simulink library "sm_aileron_actuator_mech_lib"  (R2019a)
settings: Solver=ode45  StartTime=0.0  StopTime=10.0  RelTol=1e-3
undefined symbols (not defined in the file): AAC_Param, actbase_x, actbase_y, smiData, X, Y, Z
libraries: sm_lib x600, fl_lib x3
(part 2 of 12)

== system sm_aileron_actuator_mech_lib/Aileron_Att_1/MountR_Att_1/Bracket C ==
  AilBrk_C_1_RIGID : Subsystem
  Bolt CBrk : Subsystem
  Screws CBrk : Subsystem
  Ail : PMIOPort  Side=Right
  Act : PMIOPort  Port=2  Side=Left
  connections:
  AilBrk_C_1_RIGID/LConn2 -- Act/RConn1
  AilBrk_C_1_RIGID/RConn1 -- Ail/RConn1
  Bolt CBrk/LConn1 -- Screws CBrk/LConn1 -- AilBrk_C_1_RIGID/LConn1

== system sm_aileron_actuator_mech_lib/Aileron_Att_1/MountR_Att_1/Bracket L ==
  AilBrk_L_1_RIGID : Subsystem
  Bolt LBrk : Subsystem
  Screws LBrk : Subsystem
  Ail : PMIOPort  Side=Right
  connections:
  AilBrk_L_1_RIGID/RConn1 -- Ail/RConn1
  Bolt LBrk/LConn1 -- AilBrk_L_1_RIGID/LConn1 -- Screws LBrk/LConn1

== system sm_aileron_actuator_mech_lib/Aileron_Att_1/MountR_Att_1/Bracket R ==
  AilBrk_R_1_RIGID : Subsystem
  Bolt RBrk : Subsystem
  Screws RBrk : Subsystem
  Ail : PMIOPort  Side=Right
  connections:
  AilBrk_R_1_RIGID/RConn1 -- Ail/RConn1
  Bolt RBrk/LConn1 -- AilBrk_R_1_RIGID/LConn1 -- Screws RBrk/LConn1

== system sm_aileron_actuator_mech_lib/Aileron Mech/Aileron_Att_1/MountC_Att_1/Bracket C ==
  AilBrk_C_1_RIGID : Subsystem
  Bolt CBrk : Subsystem
  Screws CBrk : Subsystem
  Ail : PMIOPort  Side=Right
  Act : PMIOPort  Port=2  Side=Left
  connections:
  AilBrk_C_1_RIGID/LConn1 -- Screws CBrk/LConn1 -- Bolt CBrk/LConn1
  AilBrk_C_1_RIGID/RConn1 -- Ail/RConn1
  AilBrk_C_1_RIGID/LConn2 -- Act/RConn1

== system sm_aileron_actuator_mech_lib/Aileron Mech/Aileron_Att_1/MountC_Att_1/Bracket L ==
  AilBrk_L_1_RIGID : Subsystem
  Bolt LBrk : Subsystem
  Screws LBrk : Subsystem
  M : PMIOPort  Side=Left
  Ail : PMIOPort  Port=2  Side=Right
  connections:
  Screws LBrk/LConn1 -- Bolt LBrk/LConn2 -- AilBrk_L_1_RIGID/LConn1
  Bolt LBrk/LConn1 -- M/RConn1
  AilBrk_L_1_RIGID/RConn1 -- Ail/RConn1

== system sm_aileron_actuator_mech_lib/Aileron Mech/Aileron_Att_1/MountC_Att_1/Bracket R ==
  AilBrk_R_1_RIGID : Subsystem
  Bolt RBrk : Subsystem
  Screws RBrk : Subsystem
  Ail : PMIOPort  Side=Right
  connections:
  AilBrk_R_1_RIGID/LConn1 -- Screws RBrk/LConn1 -- Bolt RBrk/LConn1
  AilBrk_R_1_RIGID/RConn1 -- Ail/RConn1

== system sm_aileron_actuator_mech_lib/Aileron Mech/Aileron_Att_1/MountL_Att_1/Bracket C ==
  AilBrk_C_1_RIGID : Subsystem
  Bolt CBrk : Subsystem
  Screws CBrk : Subsystem
  Ail : PMIOPort  Side=Right
  Act : PMIOPort  Port=2  Side=Left
  connections:
  AilBrk_C_1_RIGID/LConn1 -- Screws CBrk/LConn1 -- Bolt CBrk/LConn1
  AilBrk_C_1_RIGID/LConn2 -- Act/RConn1
  AilBrk_C_1_RIGID/RConn1 -- Ail/RConn1

== system sm_aileron_actuator_mech_lib/Aileron Mech/Aileron_Att_1/MountL_Att_1/Bracket L ==
  AilBrk_L_1_RIGID : Subsystem
  Bolt LBrk : Subsystem
  "Screws LBrk " : Subsystem
  Ail : PMIOPort  Side=Right
  connections:
  AilBrk_L_1_RIGID/LConn1 -- "Screws LBrk "/LConn1 -- Bolt LBrk/LConn1
  AilBrk_L_1_RIGID/RConn1 -- Ail/RConn1

== system sm_aileron_actuator_mech_lib/Aileron Mech/Aileron_Att_1/MountL_Att_1/Bracket R ==
  AilBrk_R_1_RIGID : Subsystem
  Bolt RBrk : Subsystem
  Screws RBrk : Subsystem
  Ail : PMIOPort  Side=Right
  connections:
  AilBrk_R_1_RIGID/LConn1 -- Screws RBrk/LConn1 -- Bolt RBrk/LConn1
  AilBrk_R_1_RIGID/RConn1 -- Ail/RConn1

== system sm_aileron_actuator_mech_lib/Aileron Mech/Aileron_Att_1/MountR_Att_1/Bracket C ==
  AilBrk_C_1_RIGID : Subsystem
  Bolt CBrk : Subsystem
  Screws CBrk : Subsystem
  Ail : PMIOPort  Side=Right
  Act : PMIOPort  Port=2  Side=Left
  connections:
  AilBrk_C_1_RIGID/LConn1 -- Screws CBrk/LConn1 -- Bolt CBrk/LConn1
  AilBrk_C_1_RIGID/RConn1 -- Ail/RConn1
  AilBrk_C_1_RIGID/LConn2 -- Act/RConn1

== system sm_aileron_actuator_mech_lib/Aileron Mech/Aileron_Att_1/MountR_Att_1/Bracket L ==
  AilBrk_L_1_RIGID : Subsystem
  Bolt LBrk : Subsystem
  Screws LBrk : Subsystem
  Ail : PMIOPort  Side=Right
  connections:
  Screws LBrk/LConn1 -- AilBrk_L_1_RIGID/LConn1 -- Bolt LBrk/LConn1
  AilBrk_L_1_RIGID/RConn1 -- Ail/RConn1

== system sm_aileron_actuator_mech_lib/Aileron Mech/Aileron_Att_1/MountR_Att_1/Bracket R ==
  AilBrk_R_1_RIGID : Subsystem
  Bolt RBrk : Subsystem
  Screws RBrk : Subsystem
  Ail : PMIOPort  Side=Right
  connections:
  Screws RBrk/LConn1 -- AilBrk_R_1_RIGID/LConn1 -- Bolt RBrk/LConn1
  AilBrk_R_1_RIGID/RConn1 -- Ail/RConn1

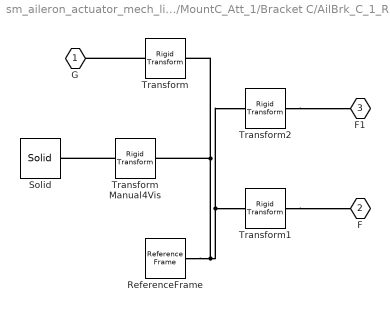
== system sm_aileron_actuator_mech_lib/Aileron_Att_1/MountC_Att_1/Bracket C/AilBrk_C_1_RIGID ==
  ReferenceFrame : sm_lib/Frames and Transforms/Reference Frame
  Solid : sm_lib/Body Elements/Solid  InertiaType=Custom  Mass=smiData.Solid(15).mass  MassUnits=kg  CenterOfMass=smiData.Solid(15).CoM  CenterOfMassUnits=m  MomentsOfInertia=smiData.Solid(15).MoI  MomentsOfInertiaUnits=kg*m^2  ProductsOfInertia=smiData.Solid(15).PoI  ProductsOfInertiaUnits=kg*m^2  BasedOnType=Density  Density=1000  DensityUnits=kg/m^3  DoExposeReferenceFrame=on  SerializedFrames=<Frames/>  GraphicType=FromGeometry  MarkerShape=Sphere  MarkerSize=10  GraphicVisPropType=SimpleVisualProperties  GraphicDiffuseColor=smiData.Solid(15).color  GraphicSpecularColor=[0.5 0.5 0.5 1.0]  GraphicAmbientColor=[0.15 0.15 0.15 1.0]  GraphicEmissiveColor=[0.0 0.0 0.0 1.0]  GraphicShininess=75  GraphicOpacity=smiData.Solid(15).opacity  GeometryShape=FromFile  RectangleSize=[1 1]  RectangleSizeUnits=m  BrickDimensions=[1 1 1]  BrickDimensionUnits=m  CylinderRadius=1  CylinderRadiusUnits=m  CylinderLength=1  CylinderLengthUnits=m  SphereRadius=1  SphereRadiusUnits=m  EllipsoidRadii=[1 1 1]  EllipsoidRadiiUnits=m  ExtrusionCrossSection=[1 1; -1 1; -1 -1; 1 -1]  ExtrusionCrossSectionUnits=m  ExtrusionLength=1  ExtrusionLengthUnits=m  PolygonNumSides=3  PolygonOuterRadius=1  PolygonOuterRadiusUnits=m  ExtGeomFileType=STEP  ExtGeomFileName=AilBrk_C.step  ExtGeomFileUnits=m  RevolutionCrossSection=[1 1; 1 -1; 2 -1; 2 1]  RevolutionCrossSectionUnits=m  RevolutionExtent=Full  RevolutionAngle=180  RevolutionAngleUnits=deg
  Transform : sm_lib/Frames and Transforms/Rigid Transform  TranslationMethod=Cartesian  TranslationStandardOffset=0  TranslationLengthUnit=m  TranslationStandardAxis=+Z  TranslationCartesianOffset=smiData.RigidTransform(98).translation  TranslationROffset=0  TranslationROffsetUnits=m  TranslationZOffset=0  TranslationZOffsetUnits=m  TranslationThetaOffset=0  TranslationThetaOffsetUnits=deg  RotationMethod=ArbitraryAxis  RotationAngleUnits=rad  RotationStandardAxis=+Z  RotationAngle=smiData.RigidTransform(98).angle  RotationArbitraryAxis=smiData.RigidTransform(98).axis  FollAlignAxisA=+X  BaseAlignAxisA=+Y  FollAlignAxisB=+Y  BaseAlignAxisB=+Z  RotationSequenceAxes=FollowerAxes  RotationSequence=XYX  RotationSequenceAngles=[0 0 0]  RotationSequenceAnglesUnits=deg  RotationMatrix=[1 0 0; 0 1 0; 0 0 1]
  Transform Manual4Vis : sm_lib/Frames and Transforms/Rigid Transform  TranslationMethod=Cartesian  TranslationStandardOffset=0  TranslationLengthUnit=m  TranslationStandardAxis=+Z  TranslationCartesianOffset=[-1 1 0]*AAC_Param.AilBrk.LRManual4Vis  TranslationROffset=0  TranslationROffsetUnits=m  TranslationZOffset=0  TranslationZOffsetUnits=m  TranslationThetaOffset=0  TranslationThetaOffsetUnits=deg  RotationMethod=None  RotationAngleUnits=deg  RotationStandardAxis=+Z  RotationAngle=0.0  RotationArbitraryAxis=[0 0 1]  FollAlignAxisA=+X  BaseAlignAxisA=+Y  FollAlignAxisB=+Y  BaseAlignAxisB=+Z  RotationSequenceAxes=FollowerAxes  RotationSequence=XYX  RotationSequenceAngles=[0 0 0]  RotationSequenceAnglesUnits=deg  RotationMatrix=[1 0 0; 0 1 0; 0 0 1]
  Transform1 : sm_lib/Frames and Transforms/Rigid Transform  TranslationMethod=Cartesian  TranslationStandardOffset=0  TranslationLengthUnit=m  TranslationStandardAxis=+Z  TranslationCartesianOffset=smiData.RigidTransform(172).translation  TranslationROffset=0  TranslationROffsetUnits=m  TranslationZOffset=0  TranslationZOffsetUnits=m  TranslationThetaOffset=0  TranslationThetaOffsetUnits=deg  RotationMethod=ArbitraryAxis  RotationAngleUnits=rad  RotationStandardAxis=+Z  RotationAngle=smiData.RigidTransform(172).angle  RotationArbitraryAxis=smiData.RigidTransform(172).axis  FollAlignAxisA=+X  BaseAlignAxisA=+Y  FollAlignAxisB=+Y  BaseAlignAxisB=+Z  RotationSequenceAxes=FollowerAxes  RotationSequence=XYX  RotationSequenceAngles=[0 0 0]  RotationSequenceAnglesUnits=deg  RotationMatrix=[1 0 0; 0 1 0; 0 0 1]
  Transform2 : sm_lib/Frames and Transforms/Rigid Transform  TranslationMethod=Cartesian  TranslationStandardOffset=0  TranslationLengthUnit=m  TranslationStandardAxis=+Z  TranslationCartesianOffset=smiData.RigidTransform(200).translation  TranslationROffset=0  TranslationROffsetUnits=m  TranslationZOffset=0  TranslationZOffsetUnits=m  TranslationThetaOffset=0  TranslationThetaOffsetUnits=deg  RotationMethod=ArbitraryAxis  RotationAngleUnits=rad  RotationStandardAxis=+Z  RotationAngle=smiData.RigidTransform(200).angle  RotationArbitraryAxis=smiData.RigidTransform(200).axis  FollAlignAxisA=+X  BaseAlignAxisA=+Y  FollAlignAxisB=+Y  BaseAlignAxisB=+Z  RotationSequenceAxes=FollowerAxes  RotationSequence=XYX  RotationSequenceAngles=[0 0 0]  RotationSequenceAnglesUnits=deg  RotationMatrix=[1 0 0; 0 1 0; 0 0 1]
  G : PMIOPort  Side=Left
  F : PMIOPort  Port=2  Side=Right
  F1 : PMIOPort  Port=3  Side=Left
  connections:
  Transform/RConn1 -- Transform Manual4Vis/LConn1 -- Transform2/LConn1 -- Transform1/LConn1 -- ReferenceFrame/RConn1
  Transform2/RConn1 -- F1/RConn1
  Transform1/RConn1 -- F/RConn1
  Transform/LConn1 -- G/RConn1
  Transform Manual4Vis/RConn1 -- Solid/RConn1

== system sm_aileron_actuator_mech_lib/Aileron_Att_1/MountC_Att_1/Bracket C/Bolt CBrk ==
  Hex_Flange_Screw_M6_1_RIGID : Subsystem
  Hex_Flange_Screw_M6_2_RIGID : Subsystem
  Hex_Flange_Screw_M6_3_RIGID : Subsystem
  Hex_Flange_Screw_M6_4_RIGID : Subsystem
  Hex_Flange_Screw_M6_5_RIGID : Subsystem
  Hex_Flange_Screw_M6_6_RIGID : Subsystem
  G : PMIOPort  Side=Left
  connections:
  Hex_Flange_Screw_M6_4_RIGID/LConn1 -- Hex_Flange_Screw_M6_3_RIGID/LConn1 -- Hex_Flange_Screw_M6_2_RIGID/LConn1 -- Hex_Flange_Screw_M6_1_RIGID/LConn1 -- G/RConn1 -- Hex_Flange_Screw_M6_5_RIGID/LConn1 -- Hex_Flange_Screw_M6_6_RIGID/LConn1

== system sm_aileron_actuator_mech_lib/Aileron_Att_1/MountC_Att_1/Bracket C/Screws CBrk ==
  Hex_Bolt_M10_3_RIGID : Subsystem
  Hex_Flange_Nut_M10_1_RIGID : Subsystem
  Washer_3_RIGID : Subsystem
  Washer_4_RIGID : Subsystem
  G : PMIOPort  Side=Left
  connections:
  Hex_Flange_Nut_M10_1_RIGID/LConn1 -- Washer_3_RIGID/LConn1 -- Washer_4_RIGID/LConn1 -- G/RConn1 -- Hex_Bolt_M10_3_RIGID/LConn1

== system sm_aileron_actuator_mech_lib/Aileron_Att_1/MountC_Att_1/Bracket L/AilBrk_L_1_RIGID ==
  ReferenceFrame : sm_lib/Frames and Transforms/Reference Frame
  Solid : sm_lib/Body Elements/Solid  InertiaType=Custom  Mass=smiData.Solid(13).mass  MassUnits=kg  CenterOfMass=smiData.Solid(13).CoM  CenterOfMassUnits=m  MomentsOfInertia=smiData.Solid(13).MoI  MomentsOfInertiaUnits=kg*m^2  ProductsOfInertia=smiData.Solid(13).PoI  ProductsOfInertiaUnits=kg*m^2  BasedOnType=Density  Density=1000  DensityUnits=kg/m^3  DoExposeReferenceFrame=on  SerializedFrames=<Frames/>  GraphicType=FromGeometry  MarkerShape=Sphere  MarkerSize=10  GraphicVisPropType=SimpleVisualProperties  GraphicDiffuseColor=smiData.Solid(13).color  GraphicSpecularColor=[0.5 0.5 0.5 1.0]  GraphicAmbientColor=[0.15 0.15 0.15 1.0]  GraphicEmissiveColor=[0.0 0.0 0.0 1.0]  GraphicShininess=75  GraphicOpacity=smiData.Solid(13).opacity  GeometryShape=FromFile  RectangleSize=[1 1]  RectangleSizeUnits=m  BrickDimensions=[1 1 1]  BrickDimensionUnits=m  CylinderRadius=1  CylinderRadiusUnits=m  CylinderLength=1  CylinderLengthUnits=m  SphereRadius=1  SphereRadiusUnits=m  EllipsoidRadii=[1 1 1]  EllipsoidRadiiUnits=m  ExtrusionCrossSection=[1 1; -1 1; -1 -1; 1 -1]  ExtrusionCrossSectionUnits=m  ExtrusionLength=1  ExtrusionLengthUnits=m  PolygonNumSides=3  PolygonOuterRadius=1  PolygonOuterRadiusUnits=m  ExtGeomFileType=STEP  ExtGeomFileName=AilBrk_L.step  ExtGeomFileUnits=m  RevolutionCrossSection=[1 1; 1 -1; 2 -1; 2 1]  RevolutionCrossSectionUnits=m  RevolutionExtent=Full  RevolutionAngle=180  RevolutionAngleUnits=deg
  Transform : sm_lib/Frames and Transforms/Rigid Transform  TranslationMethod=Cartesian  TranslationStandardOffset=0  TranslationLengthUnit=m  TranslationStandardAxis=+Z  TranslationCartesianOffset=smiData.RigidTransform(103).translation  TranslationROffset=0  TranslationROffsetUnits=m  TranslationZOffset=0  TranslationZOffsetUnits=m  TranslationThetaOffset=0  TranslationThetaOffsetUnits=deg  RotationMethod=ArbitraryAxis  RotationAngleUnits=rad  RotationStandardAxis=+Z  RotationAngle=smiData.RigidTransform(103).angle  RotationArbitraryAxis=smiData.RigidTransform(103).axis  FollAlignAxisA=+X  BaseAlignAxisA=+Y  FollAlignAxisB=+Y  BaseAlignAxisB=+Z  RotationSequenceAxes=FollowerAxes  RotationSequence=XYX  RotationSequenceAngles=[0 0 0]  RotationSequenceAnglesUnits=deg  RotationMatrix=[1 0 0; 0 1 0; 0 0 1]
  Transform Manual4Vis : sm_lib/Frames and Transforms/Rigid Transform  TranslationMethod=StandardAxis  TranslationStandardOffset=AAC_Param.AilBrk.LRManual4Vis  TranslationLengthUnit=m  TranslationStandardAxis=+Y  TranslationCartesianOffset=[0 0 0]  TranslationROffset=0  TranslationROffsetUnits=m  TranslationZOffset=0  TranslationZOffsetUnits=m  TranslationThetaOffset=0  TranslationThetaOffsetUnits=deg  RotationMethod=None  RotationAngleUnits=deg  RotationStandardAxis=+Z  RotationAngle=0.0  RotationArbitraryAxis=[0 0 1]  FollAlignAxisA=+X  BaseAlignAxisA=+Y  FollAlignAxisB=+Y  BaseAlignAxisB=+Z  RotationSequenceAxes=FollowerAxes  RotationSequence=XYX  RotationSequenceAngles=[0 0 0]  RotationSequenceAnglesUnits=deg  RotationMatrix=[1 0 0; 0 1 0; 0 0 1]
  Transform1 : sm_lib/Frames and Transforms/Rigid Transform  TranslationMethod=Cartesian  TranslationStandardOffset=0  TranslationLengthUnit=m  TranslationStandardAxis=+Z  TranslationCartesianOffset=smiData.RigidTransform(174).translation  TranslationROffset=0  TranslationROffsetUnits=m  TranslationZOffset=0  TranslationZOffsetUnits=m  TranslationThetaOffset=0  TranslationThetaOffsetUnits=deg  RotationMethod=ArbitraryAxis  RotationAngleUnits=rad  RotationStandardAxis=+Z  RotationAngle=smiData.RigidTransform(174).angle  RotationArbitraryAxis=smiData.RigidTransform(174).axis  FollAlignAxisA=+X  BaseAlignAxisA=+Y  FollAlignAxisB=+Y  BaseAlignAxisB=+Z  RotationSequenceAxes=FollowerAxes  RotationSequence=XYX  RotationSequenceAngles=[0 0 0]  RotationSequenceAnglesUnits=deg  RotationMatrix=[1 0 0; 0 1 0; 0 0 1]
  G : PMIOPort  Side=Left
  F : PMIOPort  Port=2  Side=Right
  connections:
  Transform Manual4Vis/RConn1 -- Solid/RConn1
  Transform1/RConn1 -- F/RConn1
  Transform/LConn1 -- G/RConn1
  Transform/RConn1 -- Transform1/LConn1 -- ReferenceFrame/RConn1 -- Transform Manual4Vis/LConn1

== system sm_aileron_actuator_mech_lib/Aileron_Att_1/MountC_Att_1/Bracket L/Bolt LBrk ==
  Hex_Bolt_M10_2_RIGID : Subsystem
  Washer_1_RIGID : Subsystem
  M : PMIOPort  Side=Left
  G : PMIOPort  Port=2  Side=Left
  connections:
  Washer_1_RIGID/LConn1 -- M/RConn1
  G/RConn1 -- Hex_Bolt_M10_2_RIGID/LConn1 -- Washer_1_RIGID/LConn2

== system sm_aileron_actuator_mech_lib/Aileron_Att_1/MountC_Att_1/Bracket L/Screws LBrk ==
  Oval_Head_M4_12_RIGID : Subsystem
  Oval_Head_M4_1_RIGID : Subsystem
  Oval_Head_M4_4_RIGID : Subsystem
  Oval_Head_M4_5_RIGID : Subsystem
  Oval_Head_M4_6_RIGID : Subsystem
  Oval_Head_M4_8_RIGID : Subsystem
  G : PMIOPort  Side=Left
  connections:
  Oval_Head_M4_12_RIGID/LConn1 -- Oval_Head_M4_4_RIGID/LConn1 -- Oval_Head_M4_5_RIGID/LConn1 -- Oval_Head_M4_6_RIGID/LConn1 -- Oval_Head_M4_8_RIGID/LConn1 -- G/RConn1 -- Oval_Head_M4_1_RIGID/LConn1

== system sm_aileron_actuator_mech_lib/Aileron_Att_1/MountC_Att_1/Bracket R/AilBrk_R_1_RIGID ==
  ReferenceFrame : sm_lib/Frames and Transforms/Reference Frame
  Solid : sm_lib/Body Elements/Solid  InertiaType=Custom  Mass=smiData.Solid(16).mass  MassUnits=kg  CenterOfMass=smiData.Solid(16).CoM  CenterOfMassUnits=m  MomentsOfInertia=smiData.Solid(16).MoI  MomentsOfInertiaUnits=kg*m^2  ProductsOfInertia=smiData.Solid(16).PoI  ProductsOfInertiaUnits=kg*m^2  BasedOnType=Density  Density=1000  DensityUnits=kg/m^3  DoExposeReferenceFrame=on  SerializedFrames=<Frames/>  GraphicType=FromGeometry  MarkerShape=Sphere  MarkerSize=10  GraphicVisPropType=SimpleVisualProperties  GraphicDiffuseColor=smiData.Solid(16).color  GraphicSpecularColor=[0.5 0.5 0.5 1.0]  GraphicAmbientColor=[0.15 0.15 0.15 1.0]  GraphicEmissiveColor=[0.0 0.0 0.0 1.0]  GraphicShininess=75  GraphicOpacity=smiData.Solid(16).opacity  GeometryShape=FromFile  RectangleSize=[1 1]  RectangleSizeUnits=m  BrickDimensions=[1 1 1]  BrickDimensionUnits=m  CylinderRadius=1  CylinderRadiusUnits=m  CylinderLength=1  CylinderLengthUnits=m  SphereRadius=1  SphereRadiusUnits=m  EllipsoidRadii=[1 1 1]  EllipsoidRadiiUnits=m  ExtrusionCrossSection=[1 1; -1 1; -1 -1; 1 -1]  ExtrusionCrossSectionUnits=m  ExtrusionLength=1  ExtrusionLengthUnits=m  PolygonNumSides=3  PolygonOuterRadius=1  PolygonOuterRadiusUnits=m  ExtGeomFileType=STEP  ExtGeomFileName=AilBrk_R.step  ExtGeomFileUnits=m  RevolutionCrossSection=[1 1; 1 -1; 2 -1; 2 1]  RevolutionCrossSectionUnits=m  RevolutionExtent=Full  RevolutionAngle=180  RevolutionAngleUnits=deg
  Transform : sm_lib/Frames and Transforms/Rigid Transform  TranslationMethod=Cartesian  TranslationStandardOffset=0  TranslationLengthUnit=m  TranslationStandardAxis=+Z  TranslationCartesianOffset=smiData.RigidTransform(82).translation  TranslationROffset=0  TranslationROffsetUnits=m  TranslationZOffset=0  TranslationZOffsetUnits=m  TranslationThetaOffset=0  TranslationThetaOffsetUnits=deg  RotationMethod=ArbitraryAxis  RotationAngleUnits=rad  RotationStandardAxis=+Z  RotationAngle=smiData.RigidTransform(82).angle  RotationArbitraryAxis=smiData.RigidTransform(82).axis  FollAlignAxisA=+X  BaseAlignAxisA=+Y  FollAlignAxisB=+Y  BaseAlignAxisB=+Z  RotationSequenceAxes=FollowerAxes  RotationSequence=XYX  RotationSequenceAngles=[0 0 0]  RotationSequenceAnglesUnits=deg  RotationMatrix=[1 0 0; 0 1 0; 0 0 1]
  Transform Manual4Vis : sm_lib/Frames and Transforms/Rigid Transform  TranslationMethod=StandardAxis  TranslationStandardOffset=AAC_Param.AilBrk.LRManual4Vis  TranslationLengthUnit=m  TranslationStandardAxis=-Y  TranslationCartesianOffset=[0 0 0]  TranslationROffset=0  TranslationROffsetUnits=m  TranslationZOffset=0  TranslationZOffsetUnits=m  TranslationThetaOffset=0  TranslationThetaOffsetUnits=deg  RotationMethod=None  RotationAngleUnits=deg  RotationStandardAxis=+Z  RotationAngle=0.0  RotationArbitraryAxis=[0 0 1]  FollAlignAxisA=+X  BaseAlignAxisA=+Y  FollAlignAxisB=+Y  BaseAlignAxisB=+Z  RotationSequenceAxes=FollowerAxes  RotationSequence=XYX  RotationSequenceAngles=[0 0 0]  RotationSequenceAnglesUnits=deg  RotationMatrix=[1 0 0; 0 1 0; 0 0 1]
  Transform1 : sm_lib/Frames and Transforms/Rigid Transform  TranslationMethod=Cartesian  TranslationStandardOffset=0  TranslationLengthUnit=m  TranslationStandardAxis=+Z  TranslationCartesianOffset=smiData.RigidTransform(176).translation  TranslationROffset=0  TranslationROffsetUnits=m  TranslationZOffset=0  TranslationZOffsetUnits=m  TranslationThetaOffset=0  TranslationThetaOffsetUnits=deg  RotationMethod=ArbitraryAxis  RotationAngleUnits=rad  RotationStandardAxis=+Z  RotationAngle=smiData.RigidTransform(176).angle  RotationArbitraryAxis=smiData.RigidTransform(176).axis  FollAlignAxisA=+X  BaseAlignAxisA=+Y  FollAlignAxisB=+Y  BaseAlignAxisB=+Z  RotationSequenceAxes=FollowerAxes  RotationSequence=XYX  RotationSequenceAngles=[0 0 0]  RotationSequenceAnglesUnits=deg  RotationMatrix=[1 0 0; 0 1 0; 0 0 1]
  G : PMIOPort  Side=Left
  F : PMIOPort  Port=2  Side=Right
  connections:
  Transform Manual4Vis/RConn1 -- Solid/RConn1
  Transform1/RConn1 -- F/RConn1
  Transform/LConn1 -- G/RConn1
  Transform/RConn1 -- Transform1/LConn1 -- ReferenceFrame/RConn1 -- Transform Manual4Vis/LConn1

== system sm_aileron_actuator_mech_lib/Aileron_Att_1/MountC_Att_1/Bracket R/Bolt RBrk ==
  Hex_Bolt_M10_1_RIGID : Subsystem
  Washer_2_RIGID : Subsystem
  G : PMIOPort  Side=Left
  connections:
  Washer_2_RIGID/LConn1 -- G/RConn1 -- Hex_Bolt_M10_1_RIGID/LConn1

== system sm_aileron_actuator_mech_lib/Aileron_Att_1/MountC_Att_1/Bracket R/Screws RBrk ==
  Oval_Head_M4_10_RIGID : Subsystem
  Oval_Head_M4_11_RIGID : Subsystem
  Oval_Head_M4_2_RIGID : Subsystem
  Oval_Head_M4_3_RIGID : Subsystem
  Oval_Head_M4_7_RIGID : Subsystem
  Oval_Head_M4_9_RIGID : Subsystem
  G : PMIOPort  Side=Left
  connections:
  Oval_Head_M4_7_RIGID/LConn1 -- Oval_Head_M4_9_RIGID/LConn1 -- Oval_Head_M4_2_RIGID/LConn1 -- Oval_Head_M4_11_RIGID/LConn1 -- Oval_Head_M4_10_RIGID/LConn1 -- G/RConn1 -- Oval_Head_M4_3_RIGID/LConn1

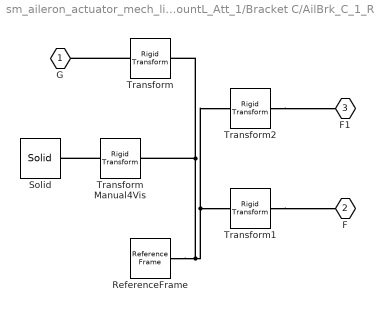
== system sm_aileron_actuator_mech_lib/Aileron_Att_1/MountL_Att_1/Bracket C/AilBrk_C_1_RIGID ==
  ReferenceFrame : sm_lib/Frames and Transforms/Reference Frame
  Solid : sm_lib/Body Elements/Solid  InertiaType=Custom  Mass=smiData.Solid(15).mass  MassUnits=kg  CenterOfMass=smiData.Solid(15).CoM  CenterOfMassUnits=m  MomentsOfInertia=smiData.Solid(15).MoI  MomentsOfInertiaUnits=kg*m^2  ProductsOfInertia=smiData.Solid(15).PoI  ProductsOfInertiaUnits=kg*m^2  BasedOnType=Density  Density=1000  DensityUnits=kg/m^3  DoExposeReferenceFrame=on  SerializedFrames=<Frames/>  GraphicType=FromGeometry  MarkerShape=Sphere  MarkerSize=10  GraphicVisPropType=SimpleVisualProperties  GraphicDiffuseColor=smiData.Solid(15).color  GraphicSpecularColor=[0.5 0.5 0.5 1.0]  GraphicAmbientColor=[0.15 0.15 0.15 1.0]  GraphicEmissiveColor=[0.0 0.0 0.0 1.0]  GraphicShininess=75  GraphicOpacity=smiData.Solid(15).opacity  GeometryShape=FromFile  RectangleSize=[1 1]  RectangleSizeUnits=m  BrickDimensions=[1 1 1]  BrickDimensionUnits=m  CylinderRadius=1  CylinderRadiusUnits=m  CylinderLength=1  CylinderLengthUnits=m  SphereRadius=1  SphereRadiusUnits=m  EllipsoidRadii=[1 1 1]  EllipsoidRadiiUnits=m  ExtrusionCrossSection=[1 1; -1 1; -1 -1; 1 -1]  ExtrusionCrossSectionUnits=m  ExtrusionLength=1  ExtrusionLengthUnits=m  PolygonNumSides=3  PolygonOuterRadius=1  PolygonOuterRadiusUnits=m  ExtGeomFileType=STEP  ExtGeomFileName=AilBrk_C.step  ExtGeomFileUnits=m  RevolutionCrossSection=[1 1; 1 -1; 2 -1; 2 1]  RevolutionCrossSectionUnits=m  RevolutionExtent=Full  RevolutionAngle=180  RevolutionAngleUnits=deg
  Transform : sm_lib/Frames and Transforms/Rigid Transform  TranslationMethod=Cartesian  TranslationStandardOffset=0  TranslationLengthUnit=m  TranslationStandardAxis=+Z  TranslationCartesianOffset=smiData.RigidTransform(161).translation  TranslationROffset=0  TranslationROffsetUnits=m  TranslationZOffset=0  TranslationZOffsetUnits=m  TranslationThetaOffset=0  TranslationThetaOffsetUnits=deg  RotationMethod=ArbitraryAxis  RotationAngleUnits=rad  RotationStandardAxis=+Z  RotationAngle=smiData.RigidTransform(161).angle  RotationArbitraryAxis=smiData.RigidTransform(161).axis  FollAlignAxisA=+X  BaseAlignAxisA=+Y  FollAlignAxisB=+Y  BaseAlignAxisB=+Z  RotationSequenceAxes=FollowerAxes  RotationSequence=XYX  RotationSequenceAngles=[0 0 0]  RotationSequenceAnglesUnits=deg  RotationMatrix=[1 0 0; 0 1 0; 0 0 1]
  Transform Manual4Vis : sm_lib/Frames and Transforms/Rigid Transform  TranslationMethod=Cartesian  TranslationStandardOffset=0  TranslationLengthUnit=m  TranslationStandardAxis=+Z  TranslationCartesianOffset=[-1 1 0]*AAC_Param.AilBrk.LRManual4Vis  TranslationROffset=0  TranslationROffsetUnits=m  TranslationZOffset=0  TranslationZOffsetUnits=m  TranslationThetaOffset=0  TranslationThetaOffsetUnits=deg  RotationMethod=None  RotationAngleUnits=deg  RotationStandardAxis=+Z  RotationAngle=0.0  RotationArbitraryAxis=[0 0 1]  FollAlignAxisA=+X  BaseAlignAxisA=+Y  FollAlignAxisB=+Y  BaseAlignAxisB=+Z  RotationSequenceAxes=FollowerAxes  RotationSequence=XYX  RotationSequenceAngles=[0 0 0]  RotationSequenceAnglesUnits=deg  RotationMatrix=[1 0 0; 0 1 0; 0 0 1]
  Transform1 : sm_lib/Frames and Transforms/Rigid Transform  TranslationMethod=Cartesian  TranslationStandardOffset=0  TranslationLengthUnit=m  TranslationStandardAxis=+Z  TranslationCartesianOffset=smiData.RigidTransform(185).translation  TranslationROffset=0  TranslationROffsetUnits=m  TranslationZOffset=0  TranslationZOffsetUnits=m  TranslationThetaOffset=0  TranslationThetaOffsetUnits=deg  RotationMethod=ArbitraryAxis  RotationAngleUnits=rad  RotationStandardAxis=+Z  RotationAngle=smiData.RigidTransform(185).angle  RotationArbitraryAxis=smiData.RigidTransform(185).axis  FollAlignAxisA=+X  BaseAlignAxisA=+Y  FollAlignAxisB=+Y  BaseAlignAxisB=+Z  RotationSequenceAxes=FollowerAxes  RotationSequence=XYX  RotationSequenceAngles=[0 0 0]  RotationSequenceAnglesUnits=deg  RotationMatrix=[1 0 0; 0 1 0; 0 0 1]
  Transform2 : sm_lib/Frames and Transforms/Rigid Transform  TranslationMethod=Cartesian  TranslationStandardOffset=0  TranslationLengthUnit=m  TranslationStandardAxis=+Z  TranslationCartesianOffset=smiData.RigidTransform(202).translation  TranslationROffset=0  TranslationROffsetUnits=m  TranslationZOffset=0  TranslationZOffsetUnits=m  TranslationThetaOffset=0  TranslationThetaOffsetUnits=deg  RotationMethod=ArbitraryAxis  RotationAngleUnits=rad  RotationStandardAxis=+Z  RotationAngle=smiData.RigidTransform(202).angle  RotationArbitraryAxis=smiData.RigidTransform(202).axis  FollAlignAxisA=+X  BaseAlignAxisA=+Y  FollAlignAxisB=+Y  BaseAlignAxisB=+Z  RotationSequenceAxes=FollowerAxes  RotationSequence=XYX  RotationSequenceAngles=[0 0 0]  RotationSequenceAnglesUnits=deg  RotationMatrix=[1 0 0; 0 1 0; 0 0 1]
  G : PMIOPort  Side=Left
  F : PMIOPort  Port=2  Side=Right
  F1 : PMIOPort  Port=3  Side=Left
  connections:
  Transform Manual4Vis/RConn1 -- Solid/RConn1
  Transform2/RConn1 -- F1/RConn1
  Transform1/RConn1 -- F/RConn1
  Transform/LConn1 -- G/RConn1
  Transform/RConn1 -- Transform2/LConn1 -- Transform1/LConn1 -- ReferenceFrame/RConn1 -- Transform Manual4Vis/LConn1

== system sm_aileron_actuator_mech_lib/Aileron_Att_1/MountL_Att_1/Bracket C/Bolt CBrk ==
  Hex_Bolt_M10_3_RIGID : Subsystem
  Hex_Flange_Nut_M10_1_RIGID : Subsystem
  Washer_1_RIGID : Subsystem
  Washer_4_RIGID : Subsystem
  G : PMIOPort  Side=Left
  connections:
  Washer_4_RIGID/LConn1 -- Washer_1_RIGID/LConn1 -- Hex_Bolt_M10_3_RIGID/LConn1 -- G/RConn1 -- Hex_Flange_Nut_M10_1_RIGID/LConn1

== system sm_aileron_actuator_mech_lib/Aileron_Att_1/MountL_Att_1/Bracket C/Screws CBrk ==
  Hex_Flange_Screw_M6_1_RIGID : Subsystem
  Hex_Flange_Screw_M6_2_RIGID : Subsystem
  Hex_Flange_Screw_M6_3_RIGID : Subsystem
  Hex_Flange_Screw_M6_4_RIGID : Subsystem
  Hex_Flange_Screw_M6_5_RIGID : Subsystem
  Hex_Flange_Screw_M6_6_RIGID : Subsystem
  G : PMIOPort  Side=Left
  connections:
  Hex_Flange_Screw_M6_5_RIGID/LConn1 -- Hex_Flange_Screw_M6_4_RIGID/LConn1 -- Hex_Flange_Screw_M6_3_RIGID/LConn1 -- Hex_Flange_Screw_M6_2_RIGID/LConn1 -- Hex_Flange_Screw_M6_1_RIGID/LConn1 -- G/RConn1 -- Hex_Flange_Screw_M6_6_RIGID/LConn1

== system sm_aileron_actuator_mech_lib/Aileron_Att_1/MountL_Att_1/Bracket L/AilBrk_L_1_RIGID ==
  ReferenceFrame : sm_lib/Frames and Transforms/Reference Frame
  Solid : sm_lib/Body Elements/Solid  InertiaType=Custom  Mass=smiData.Solid(13).mass  MassUnits=kg  CenterOfMass=smiData.Solid(13).CoM  CenterOfMassUnits=m  MomentsOfInertia=smiData.Solid(13).MoI  MomentsOfInertiaUnits=kg*m^2  ProductsOfInertia=smiData.Solid(13).PoI  ProductsOfInertiaUnits=kg*m^2  BasedOnType=Density  Density=1000  DensityUnits=kg/m^3  DoExposeReferenceFrame=on  SerializedFrames=<Frames/>  GraphicType=FromGeometry  MarkerShape=Sphere  MarkerSize=10  GraphicVisPropType=SimpleVisualProperties  GraphicDiffuseColor=smiData.Solid(13).color  GraphicSpecularColor=[0.5 0.5 0.5 1.0]  GraphicAmbientColor=[0.15 0.15 0.15 1.0]  GraphicEmissiveColor=[0.0 0.0 0.0 1.0]  GraphicShininess=75  GraphicOpacity=smiData.Solid(13).opacity  GeometryShape=FromFile  RectangleSize=[1 1]  RectangleSizeUnits=m  BrickDimensions=[1 1 1]  BrickDimensionUnits=m  CylinderRadius=1  CylinderRadiusUnits=m  CylinderLength=1  CylinderLengthUnits=m  SphereRadius=1  SphereRadiusUnits=m  EllipsoidRadii=[1 1 1]  EllipsoidRadiiUnits=m  ExtrusionCrossSection=[1 1; -1 1; -1 -1; 1 -1]  ExtrusionCrossSectionUnits=m  ExtrusionLength=1  ExtrusionLengthUnits=m  PolygonNumSides=3  PolygonOuterRadius=1  PolygonOuterRadiusUnits=m  ExtGeomFileType=STEP  ExtGeomFileName=AilBrk_L.step  ExtGeomFileUnits=m  RevolutionCrossSection=[1 1; 1 -1; 2 -1; 2 1]  RevolutionCrossSectionUnits=m  RevolutionExtent=Full  RevolutionAngle=180  RevolutionAngleUnits=deg
  Transform : sm_lib/Frames and Transforms/Rigid Transform  TranslationMethod=Cartesian  TranslationStandardOffset=0  TranslationLengthUnit=m  TranslationStandardAxis=+Z  TranslationCartesianOffset=smiData.RigidTransform(150).translation  TranslationROffset=0  TranslationROffsetUnits=m  TranslationZOffset=0  TranslationZOffsetUnits=m  TranslationThetaOffset=0  TranslationThetaOffsetUnits=deg  RotationMethod=ArbitraryAxis  RotationAngleUnits=rad  RotationStandardAxis=+Z  RotationAngle=smiData.RigidTransform(150).angle  RotationArbitraryAxis=smiData.RigidTransform(150).axis  FollAlignAxisA=+X  BaseAlignAxisA=+Y  FollAlignAxisB=+Y  BaseAlignAxisB=+Z  RotationSequenceAxes=FollowerAxes  RotationSequence=XYX  RotationSequenceAngles=[0 0 0]  RotationSequenceAnglesUnits=deg  RotationMatrix=[1 0 0; 0 1 0; 0 0 1]
  Transform Manual4Vis : sm_lib/Frames and Transforms/Rigid Transform  TranslationMethod=StandardAxis  TranslationStandardOffset=AAC_Param.AilBrk.LRManual4Vis  TranslationLengthUnit=m  TranslationStandardAxis=+Y  TranslationCartesianOffset=[0 0 0]  TranslationROffset=0  TranslationROffsetUnits=m  TranslationZOffset=0  TranslationZOffsetUnits=m  TranslationThetaOffset=0  TranslationThetaOffsetUnits=deg  RotationMethod=None  RotationAngleUnits=deg  RotationStandardAxis=+Z  RotationAngle=0.0  RotationArbitraryAxis=[0 0 1]  FollAlignAxisA=+X  BaseAlignAxisA=+Y  FollAlignAxisB=+Y  BaseAlignAxisB=+Z  RotationSequenceAxes=FollowerAxes  RotationSequence=XYX  RotationSequenceAngles=[0 0 0]  RotationSequenceAnglesUnits=deg  RotationMatrix=[1 0 0; 0 1 0; 0 0 1]
  Transform1 : sm_lib/Frames and Transforms/Rigid Transform  TranslationMethod=Cartesian  TranslationStandardOffset=0  TranslationLengthUnit=m  TranslationStandardAxis=+Z  TranslationCartesianOffset=smiData.RigidTransform(183).translation  TranslationROffset=0  TranslationROffsetUnits=m  TranslationZOffset=0  TranslationZOffsetUnits=m  TranslationThetaOffset=0  TranslationThetaOffsetUnits=deg  RotationMethod=ArbitraryAxis  RotationAngleUnits=rad  RotationStandardAxis=+Z  RotationAngle=smiData.RigidTransform(183).angle  RotationArbitraryAxis=smiData.RigidTransform(183).axis  FollAlignAxisA=+X  BaseAlignAxisA=+Y  FollAlignAxisB=+Y  BaseAlignAxisB=+Z  RotationSequenceAxes=FollowerAxes  RotationSequence=XYX  RotationSequenceAngles=[0 0 0]  RotationSequenceAnglesUnits=deg  RotationMatrix=[1 0 0; 0 1 0; 0 0 1]
  G : PMIOPort  Side=Left
  F : PMIOPort  Port=2  Side=Right
  connections:
  Transform Manual4Vis/RConn1 -- Solid/RConn1
  Transform1/RConn1 -- F/RConn1
  Transform/LConn1 -- G/RConn1
  Transform/RConn1 -- Transform1/LConn1 -- ReferenceFrame/RConn1 -- Transform Manual4Vis/LConn1

== system sm_aileron_actuator_mech_lib/Aileron_Att_1/MountL_Att_1/Bracket L/Bolt LBrk ==
  Hex_Bolt_M10_1_RIGID : Subsystem
  Washer_3_RIGID : Subsystem
  G : PMIOPort  Side=Left
  connections:
  Hex_Bolt_M10_1_RIGID/LConn1 -- G/RConn1 -- Washer_3_RIGID/LConn1

== system sm_aileron_actuator_mech_lib/Aileron_Att_1/MountL_Att_1/Bracket L/Screws LBrk  ==
  Oval_Head_M4_2_RIGID : Subsystem
  Oval_Head_M4_3_RIGID : Subsystem
  Oval_Head_M4_4_RIGID : Subsystem
  Oval_Head_M4_5_RIGID : Subsystem
  Oval_Head_M4_7_RIGID : Subsystem
  Oval_Head_M4_9_RIGID : Subsystem
  G : PMIOPort  Side=Left
  connections:
  Oval_Head_M4_5_RIGID/LConn1 -- Oval_Head_M4_4_RIGID/LConn1 -- Oval_Head_M4_3_RIGID/LConn1 -- Oval_Head_M4_2_RIGID/LConn1 -- G/RConn1 -- Oval_Head_M4_7_RIGID/LConn1 -- Oval_Head_M4_9_RIGID/LConn1

== system sm_aileron_actuator_mech_lib/Aileron_Att_1/MountL_Att_1/Bracket R/AilBrk_R_1_RIGID ==
  ReferenceFrame : sm_lib/Frames and Transforms/Reference Frame
  Solid : sm_lib/Body Elements/Solid  InertiaType=Custom  Mass=smiData.Solid(16).mass  MassUnits=kg  CenterOfMass=smiData.Solid(16).CoM  CenterOfMassUnits=m  MomentsOfInertia=smiData.Solid(16).MoI  MomentsOfInertiaUnits=kg*m^2  ProductsOfInertia=smiData.Solid(16).PoI  ProductsOfInertiaUnits=kg*m^2  BasedOnType=Density  Density=1000  DensityUnits=kg/m^3  DoExposeReferenceFrame=on  SerializedFrames=<Frames/>  GraphicType=FromGeometry  MarkerShape=Sphere  MarkerSize=10  GraphicVisPropType=SimpleVisualProperties  GraphicDiffuseColor=smiData.Solid(16).color  GraphicSpecularColor=[0.5 0.5 0.5 1.0]  GraphicAmbientColor=[0.15 0.15 0.15 1.0]  GraphicEmissiveColor=[0.0 0.0 0.0 1.0]  GraphicShininess=75  GraphicOpacity=smiData.Solid(16).opacity  GeometryShape=FromFile  RectangleSize=[1 1]  RectangleSizeUnits=m  BrickDimensions=[1 1 1]  BrickDimensionUnits=m  CylinderRadius=1  CylinderRadiusUnits=m  CylinderLength=1  CylinderLengthUnits=m  SphereRadius=1  SphereRadiusUnits=m  EllipsoidRadii=[1 1 1]  EllipsoidRadiiUnits=m  ExtrusionCrossSection=[1 1; -1 1; -1 -1; 1 -1]  ExtrusionCrossSectionUnits=m  ExtrusionLength=1  ExtrusionLengthUnits=m  PolygonNumSides=3  PolygonOuterRadius=1  PolygonOuterRadiusUnits=m  ExtGeomFileType=STEP  ExtGeomFileName=AilBrk_R.step  ExtGeomFileUnits=m  RevolutionCrossSection=[1 1; 1 -1; 2 -1; 2 1]  RevolutionCrossSectionUnits=m  RevolutionExtent=Full  RevolutionAngle=180  RevolutionAngleUnits=deg
  Transform : sm_lib/Frames and Transforms/Rigid Transform  TranslationMethod=Cartesian  TranslationStandardOffset=0  TranslationLengthUnit=m  TranslationStandardAxis=+Z  TranslationCartesianOffset=smiData.RigidTransform(146).translation  TranslationROffset=0  TranslationROffsetUnits=m  TranslationZOffset=0  TranslationZOffsetUnits=m  TranslationThetaOffset=0  TranslationThetaOffsetUnits=deg  RotationMethod=ArbitraryAxis  RotationAngleUnits=rad  RotationStandardAxis=+Z  RotationAngle=smiData.RigidTransform(146).angle  RotationArbitraryAxis=smiData.RigidTransform(146).axis  FollAlignAxisA=+X  BaseAlignAxisA=+Y  FollAlignAxisB=+Y  BaseAlignAxisB=+Z  RotationSequenceAxes=FollowerAxes  RotationSequence=XYX  RotationSequenceAngles=[0 0 0]  RotationSequenceAnglesUnits=deg  RotationMatrix=[1 0 0; 0 1 0; 0 0 1]
  Transform Manual4Vis : sm_lib/Frames and Transforms/Rigid Transform  TranslationMethod=StandardAxis  TranslationStandardOffset=AAC_Param.AilBrk.LRManual4Vis  TranslationLengthUnit=m  TranslationStandardAxis=-Y  TranslationCartesianOffset=[0 0 0]  TranslationROffset=0  TranslationROffsetUnits=m  TranslationZOffset=0  TranslationZOffsetUnits=m  TranslationThetaOffset=0  TranslationThetaOffsetUnits=deg  RotationMethod=None  RotationAngleUnits=deg  RotationStandardAxis=+Z  RotationAngle=0.0  RotationArbitraryAxis=[0 0 1]  FollAlignAxisA=+X  BaseAlignAxisA=+Y  FollAlignAxisB=+Y  BaseAlignAxisB=+Z  RotationSequenceAxes=FollowerAxes  RotationSequence=XYX  RotationSequenceAngles=[0 0 0]  RotationSequenceAnglesUnits=deg  RotationMatrix=[1 0 0; 0 1 0; 0 0 1]
  Transform1 : sm_lib/Frames and Transforms/Rigid Transform  TranslationMethod=Cartesian  TranslationStandardOffset=0  TranslationLengthUnit=m  TranslationStandardAxis=+Z  TranslationCartesianOffset=smiData.RigidTransform(187).translation  TranslationROffset=0  TranslationROffsetUnits=m  TranslationZOffset=0  TranslationZOffsetUnits=m  TranslationThetaOffset=0  TranslationThetaOffsetUnits=deg  RotationMethod=ArbitraryAxis  RotationAngleUnits=rad  RotationStandardAxis=+Z  RotationAngle=smiData.RigidTransform(187).angle  RotationArbitraryAxis=smiData.RigidTransform(187).axis  FollAlignAxisA=+X  BaseAlignAxisA=+Y  FollAlignAxisB=+Y  BaseAlignAxisB=+Z  RotationSequenceAxes=FollowerAxes  RotationSequence=XYX  RotationSequenceAngles=[0 0 0]  RotationSequenceAnglesUnits=deg  RotationMatrix=[1 0 0; 0 1 0; 0 0 1]
  G : PMIOPort  Side=Left
  F : PMIOPort  Port=2  Side=Right
  connections:
  Transform1/LConn1 -- Transform/RConn1 -- Transform Manual4Vis/LConn1 -- ReferenceFrame/RConn1
  Transform1/RConn1 -- F/RConn1
  Transform/LConn1 -- G/RConn1
  Transform Manual4Vis/RConn1 -- Solid/RConn1

== system sm_aileron_actuator_mech_lib/Aileron_Att_1/MountL_Att_1/Bracket R/Bolt RBrk ==
  Hex_Bolt_M10_2_RIGID : Subsystem
  Washer_2_RIGID : Subsystem
  G : PMIOPort  Side=Left
  connections:
  Hex_Bolt_M10_2_RIGID/LConn1 -- Washer_2_RIGID/LConn1 -- G/RConn1

== system sm_aileron_actuator_mech_lib/Aileron_Att_1/MountL_Att_1/Bracket R/Screws RBrk ==
  Oval_Head_M4_10_RIGID : Subsystem
  Oval_Head_M4_11_RIGID : Subsystem
  Oval_Head_M4_12_RIGID : Subsystem
  Oval_Head_M4_1_RIGID : Subsystem
  Oval_Head_M4_6_RIGID : Subsystem
  Oval_Head_M4_8_RIGID : Subsystem
  G : PMIOPort  Side=Left
  connections:
  Oval_Head_M4_8_RIGID/LConn1 -- Oval_Head_M4_1_RIGID/LConn1 -- Oval_Head_M4_12_RIGID/LConn1 -- Oval_Head_M4_11_RIGID/LConn1 -- Oval_Head_M4_10_RIGID/LConn1 -- G/RConn1 -- Oval_Head_M4_6_RIGID/LConn1

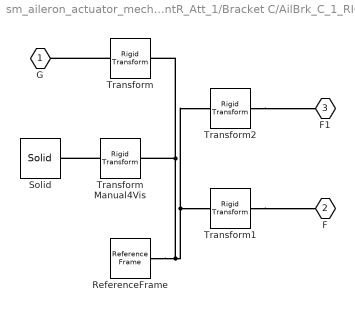
== system sm_aileron_actuator_mech_lib/Aileron_Att_1/MountR_Att_1/Bracket C/AilBrk_C_1_RIGID ==
  ReferenceFrame : sm_lib/Frames and Transforms/Reference Frame
  Solid : sm_lib/Body Elements/Solid  InertiaType=Custom  Mass=smiData.Solid(15).mass  MassUnits=kg  CenterOfMass=smiData.Solid(15).CoM  CenterOfMassUnits=m  MomentsOfInertia=smiData.Solid(15).MoI  MomentsOfInertiaUnits=kg*m^2  ProductsOfInertia=smiData.Solid(15).PoI  ProductsOfInertiaUnits=kg*m^2  BasedOnType=Density  Density=1000  DensityUnits=kg/m^3  DoExposeReferenceFrame=on  SerializedFrames=<Frames/>  GraphicType=FromGeometry  MarkerShape=Sphere  MarkerSize=10  GraphicVisPropType=SimpleVisualProperties  GraphicDiffuseColor=smiData.Solid(15).color  GraphicSpecularColor=[0.5 0.5 0.5 1.0]  GraphicAmbientColor=[0.15 0.15 0.15 1.0]  GraphicEmissiveColor=[0.0 0.0 0.0 1.0]  GraphicShininess=75  GraphicOpacity=smiData.Solid(15).opacity  GeometryShape=FromFile  RectangleSize=[1 1]  RectangleSizeUnits=m  BrickDimensions=[1 1 1]  BrickDimensionUnits=m  CylinderRadius=1  CylinderRadiusUnits=m  CylinderLength=1  CylinderLengthUnits=m  SphereRadius=1  SphereRadiusUnits=m  EllipsoidRadii=[1 1 1]  EllipsoidRadiiUnits=m  ExtrusionCrossSection=[1 1; -1 1; -1 -1; 1 -1]  ExtrusionCrossSectionUnits=m  ExtrusionLength=1  ExtrusionLengthUnits=m  PolygonNumSides=3  PolygonOuterRadius=1  PolygonOuterRadiusUnits=m  ExtGeomFileType=STEP  ExtGeomFileName=AilBrk_C.step  ExtGeomFileUnits=m  RevolutionCrossSection=[1 1; 1 -1; 2 -1; 2 1]  RevolutionCrossSectionUnits=m  RevolutionExtent=Full  RevolutionAngle=180  RevolutionAngleUnits=deg
  Transform : sm_lib/Frames and Transforms/Rigid Transform  TranslationMethod=Cartesian  TranslationStandardOffset=0  TranslationLengthUnit=m  TranslationStandardAxis=+Z  TranslationCartesianOffset=smiData.RigidTransform(136).translation  TranslationROffset=0  TranslationROffsetUnits=m  TranslationZOffset=0  TranslationZOffsetUnits=m  TranslationThetaOffset=0  TranslationThetaOffsetUnits=deg  RotationMethod=ArbitraryAxis  RotationAngleUnits=rad  RotationStandardAxis=+Z  RotationAngle=smiData.RigidTransform(136).angle  RotationArbitraryAxis=smiData.RigidTransform(136).axis  FollAlignAxisA=+X  BaseAlignAxisA=+Y  FollAlignAxisB=+Y  BaseAlignAxisB=+Z  RotationSequenceAxes=FollowerAxes  RotationSequence=XYX  RotationSequenceAngles=[0 0 0]  RotationSequenceAnglesUnits=deg  RotationMatrix=[1 0 0; 0 1 0; 0 0 1]
  Transform Manual4Vis : sm_lib/Frames and Transforms/Rigid Transform  TranslationMethod=Cartesian  TranslationStandardOffset=0  TranslationLengthUnit=m  TranslationStandardAxis=+Z  TranslationCartesianOffset=[-1 1 0]*AAC_Param.AilBrk.LRManual4Vis  TranslationROffset=0  TranslationROffsetUnits=m  TranslationZOffset=0  TranslationZOffsetUnits=m  TranslationThetaOffset=0  TranslationThetaOffsetUnits=deg  RotationMethod=None  RotationAngleUnits=deg  RotationStandardAxis=+Z  RotationAngle=0.0  RotationArbitraryAxis=[0 0 1]  FollAlignAxisA=+X  BaseAlignAxisA=+Y  FollAlignAxisB=+Y  BaseAlignAxisB=+Z  RotationSequenceAxes=FollowerAxes  RotationSequence=XYX  RotationSequenceAngles=[0 0 0]  RotationSequenceAnglesUnits=deg  RotationMatrix=[1 0 0; 0 1 0; 0 0 1]
  Transform1 : sm_lib/Frames and Transforms/Rigid Transform  TranslationMethod=Cartesian  TranslationStandardOffset=0  TranslationLengthUnit=m  TranslationStandardAxis=+Z  TranslationCartesianOffset=smiData.RigidTransform(181).translation  TranslationROffset=0  TranslationROffsetUnits=m  TranslationZOffset=0  TranslationZOffsetUnits=m  TranslationThetaOffset=0  TranslationThetaOffsetUnits=deg  RotationMethod=ArbitraryAxis  RotationAngleUnits=rad  RotationStandardAxis=+Z  RotationAngle=smiData.RigidTransform(181).angle  RotationArbitraryAxis=smiData.RigidTransform(181).axis  FollAlignAxisA=+X  BaseAlignAxisA=+Y  FollAlignAxisB=+Y  BaseAlignAxisB=+Z  RotationSequenceAxes=FollowerAxes  RotationSequence=XYX  RotationSequenceAngles=[0 0 0]  RotationSequenceAnglesUnits=deg  RotationMatrix=[1 0 0; 0 1 0; 0 0 1]
  Transform2 : sm_lib/Frames and Transforms/Rigid Transform  TranslationMethod=Cartesian  TranslationStandardOffset=0  TranslationLengthUnit=m  TranslationStandardAxis=+Z  TranslationCartesianOffset=smiData.RigidTransform(192).translation  TranslationROffset=0  TranslationROffsetUnits=m  TranslationZOffset=0  TranslationZOffsetUnits=m  TranslationThetaOffset=0  TranslationThetaOffsetUnits=deg  RotationMethod=ArbitraryAxis  RotationAngleUnits=rad  RotationStandardAxis=+Z  RotationAngle=smiData.RigidTransform(192).angle  RotationArbitraryAxis=smiData.RigidTransform(192).axis  FollAlignAxisA=+X  BaseAlignAxisA=+Y  FollAlignAxisB=+Y  BaseAlignAxisB=+Z  RotationSequenceAxes=FollowerAxes  RotationSequence=XYX  RotationSequenceAngles=[0 0 0]  RotationSequenceAnglesUnits=deg  RotationMatrix=[1 0 0; 0 1 0; 0 0 1]
  G : PMIOPort  Side=Left
  F : PMIOPort  Port=2  Side=Right
  F1 : PMIOPort  Port=3  Side=Left
  connections:
  Transform Manual4Vis/RConn1 -- Solid/RConn1
  Transform2/RConn1 -- F1/RConn1
  Transform1/RConn1 -- F/RConn1
  Transform/LConn1 -- G/RConn1
  Transform/RConn1 -- Transform2/LConn1 -- Transform1/LConn1 -- ReferenceFrame/RConn1 -- Transform Manual4Vis/LConn1

== system sm_aileron_actuator_mech_lib/Aileron_Att_1/MountR_Att_1/Bracket C/Bolt CBrk ==
  Hex_Bolt_M10_3_RIGID : Subsystem
  Hex_Flange_Nut_M10_1_RIGID : Subsystem
  Washer_2_RIGID : Subsystem
  Washer_4_RIGID : Subsystem
  B : PMIOPort  Side=Left
  connections:
  Hex_Bolt_M10_3_RIGID/LConn1 -- Hex_Flange_Nut_M10_1_RIGID/LConn1 -- Washer_2_RIGID/LConn1 -- B/RConn1 -- Washer_4_RIGID/LConn1

== system sm_aileron_actuator_mech_lib/Aileron_Att_1/MountR_Att_1/Bracket C/Screws CBrk ==
  Hex_Flange_Screw_M6_1_RIGID : Subsystem
  Hex_Flange_Screw_M6_2_RIGID : Subsystem
  Hex_Flange_Screw_M6_3_RIGID : Subsystem
  Hex_Flange_Screw_M6_4_RIGID : Subsystem
  Hex_Flange_Screw_M6_5_RIGID : Subsystem
  Hex_Flange_Screw_M6_6_RIGID : Subsystem
  B : PMIOPort  Side=Left
  connections:
  Hex_Flange_Screw_M6_1_RIGID/LConn1 -- Hex_Flange_Screw_M6_2_RIGID/LConn1 -- Hex_Flange_Screw_M6_3_RIGID/LConn1 -- Hex_Flange_Screw_M6_4_RIGID/LConn1 -- Hex_Flange_Screw_M6_5_RIGID/LConn1 -- Hex_Flange_Screw_M6_6_RIGID/LConn1 -- B/RConn1

== system sm_aileron_actuator_mech_lib/Aileron_Att_1/MountR_Att_1/Bracket L/AilBrk_L_1_RIGID ==
  ReferenceFrame : sm_lib/Frames and Transforms/Reference Frame
  Solid : sm_lib/Body Elements/Solid  InertiaType=Custom  Mass=smiData.Solid(13).mass  MassUnits=kg  CenterOfMass=smiData.Solid(13).CoM  CenterOfMassUnits=m  MomentsOfInertia=smiData.Solid(13).MoI  MomentsOfInertiaUnits=kg*m^2  ProductsOfInertia=smiData.Solid(13).PoI  ProductsOfInertiaUnits=kg*m^2  BasedOnType=Density  Density=1000  DensityUnits=kg/m^3  DoExposeReferenceFrame=on  SerializedFrames=<Frames/>  GraphicType=FromGeometry  MarkerShape=Sphere  MarkerSize=10  GraphicVisPropType=SimpleVisualProperties  GraphicDiffuseColor=smiData.Solid(13).color  GraphicSpecularColor=[0.5 0.5 0.5 1.0]  GraphicAmbientColor=[0.15 0.15 0.15 1.0]  GraphicEmissiveColor=[0.0 0.0 0.0 1.0]  GraphicShininess=75  GraphicOpacity=smiData.Solid(13).opacity  GeometryShape=FromFile  RectangleSize=[1 1]  RectangleSizeUnits=m  BrickDimensions=[1 1 1]  BrickDimensionUnits=m  CylinderRadius=1  CylinderRadiusUnits=m  CylinderLength=1  CylinderLengthUnits=m  SphereRadius=1  SphereRadiusUnits=m  EllipsoidRadii=[1 1 1]  EllipsoidRadiiUnits=m  ExtrusionCrossSection=[1 1; -1 1; -1 -1; 1 -1]  ExtrusionCrossSectionUnits=m  ExtrusionLength=1  ExtrusionLengthUnits=m  PolygonNumSides=3  PolygonOuterRadius=1  PolygonOuterRadiusUnits=m  ExtGeomFileType=STEP  ExtGeomFileName=AilBrk_L.step  ExtGeomFileUnits=m  RevolutionCrossSection=[1 1; 1 -1; 2 -1; 2 1]  RevolutionCrossSectionUnits=m  RevolutionExtent=Full  RevolutionAngle=180  RevolutionAngleUnits=deg
  Transform : sm_lib/Frames and Transforms/Rigid Transform  TranslationMethod=Cartesian  TranslationStandardOffset=0  TranslationLengthUnit=m  TranslationStandardAxis=+Z  TranslationCartesianOffset=smiData.RigidTransform(116).translation  TranslationROffset=0  TranslationROffsetUnits=m  TranslationZOffset=0  TranslationZOffsetUnits=m  TranslationThetaOffset=0  TranslationThetaOffsetUnits=deg  RotationMethod=ArbitraryAxis  RotationAngleUnits=rad  RotationStandardAxis=+Z  RotationAngle=smiData.RigidTransform(116).angle  RotationArbitraryAxis=smiData.RigidTransform(116).axis  FollAlignAxisA=+X  BaseAlignAxisA=+Y  FollAlignAxisB=+Y  BaseAlignAxisB=+Z  RotationSequenceAxes=FollowerAxes  RotationSequence=XYX  RotationSequenceAngles=[0 0 0]  RotationSequenceAnglesUnits=deg  RotationMatrix=[1 0 0; 0 1 0; 0 0 1]
  Transform Manual4Vis : sm_lib/Frames and Transforms/Rigid Transform  TranslationMethod=StandardAxis  TranslationStandardOffset=AAC_Param.AilBrk.LRManual4Vis  TranslationLengthUnit=m  TranslationStandardAxis=+Y  TranslationCartesianOffset=[0 0 0]  TranslationROffset=0  TranslationROffsetUnits=m  TranslationZOffset=0  TranslationZOffsetUnits=m  TranslationThetaOffset=0  TranslationThetaOffsetUnits=deg  RotationMethod=None  RotationAngleUnits=deg  RotationStandardAxis=+Z  RotationAngle=0.0  RotationArbitraryAxis=[0 0 1]  FollAlignAxisA=+X  BaseAlignAxisA=+Y  FollAlignAxisB=+Y  BaseAlignAxisB=+Z  RotationSequenceAxes=FollowerAxes  RotationSequence=XYX  RotationSequenceAngles=[0 0 0]  RotationSequenceAnglesUnits=deg  RotationMatrix=[1 0 0; 0 1 0; 0 0 1]
  Transform1 : sm_lib/Frames and Transforms/Rigid Transform  TranslationMethod=Cartesian  TranslationStandardOffset=0  TranslationLengthUnit=m  TranslationStandardAxis=+Z  TranslationCartesianOffset=smiData.RigidTransform(179).translation  TranslationROffset=0  TranslationROffsetUnits=m  TranslationZOffset=0  TranslationZOffsetUnits=m  TranslationThetaOffset=0  TranslationThetaOffsetUnits=deg  RotationMethod=ArbitraryAxis  RotationAngleUnits=rad  RotationStandardAxis=+Z  RotationAngle=smiData.RigidTransform(179).angle  RotationArbitraryAxis=smiData.RigidTransform(179).axis  FollAlignAxisA=+X  BaseAlignAxisA=+Y  FollAlignAxisB=+Y  BaseAlignAxisB=+Z  RotationSequenceAxes=FollowerAxes  RotationSequence=XYX  RotationSequenceAngles=[0 0 0]  RotationSequenceAnglesUnits=deg  RotationMatrix=[1 0 0; 0 1 0; 0 0 1]
  G : PMIOPort  Side=Left
  F : PMIOPort  Port=2  Side=Right
  connections:
  Transform Manual4Vis/RConn1 -- Solid/RConn1
  Transform1/RConn1 -- F/RConn1
  Transform/LConn1 -- G/RConn1
  Transform/RConn1 -- Transform1/LConn1 -- ReferenceFrame/RConn1 -- Transform Manual4Vis/LConn1

== system sm_aileron_actuator_mech_lib/Aileron_Att_1/MountR_Att_1/Bracket L/Bolt LBrk ==
  Hex_Bolt_M10_1_RIGID : Subsystem
  Washer_1_RIGID : Subsystem
  B : PMIOPort  Side=Left
  connections:
  Hex_Bolt_M10_1_RIGID/LConn1 -- Washer_1_RIGID/LConn1 -- B/RConn1

== system sm_aileron_actuator_mech_lib/Aileron_Att_1/MountR_Att_1/Bracket L/Screws LBrk ==
  Oval_Head_M4_10_RIGID : Subsystem
  Oval_Head_M4_11_RIGID : Subsystem
  Oval_Head_M4_12_RIGID : Subsystem
  Oval_Head_M4_5_RIGID : Subsystem
  Oval_Head_M4_6_RIGID : Subsystem
  Oval_Head_M4_8_RIGID : Subsystem
  B : PMIOPort  Side=Left
  connections:
  B/RConn1 -- Oval_Head_M4_8_RIGID/LConn1 -- Oval_Head_M4_6_RIGID/LConn1 -- Oval_Head_M4_5_RIGID/LConn1 -- Oval_Head_M4_11_RIGID/LConn1 -- Oval_Head_M4_12_RIGID/LConn1 -- Oval_Head_M4_10_RIGID/LConn1
